simulink model "IMTrialSensorFinal"  (R2023b)
settings: Solver=VariableStepAuto  StartTime=0.0  StopTime=14  FixedStep=10e-6  RelTol=1e-3
settings Model: Creator=Aryasetya  LastModifiedBy=Aryasetya
settings ModelReferenceCC: EnableRefExpFcnMdlSchedulingChecks=on

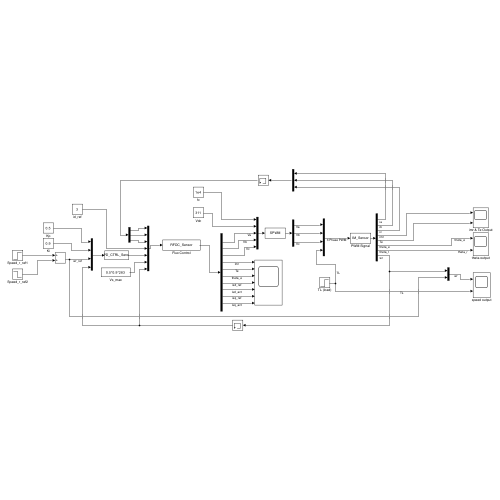
[thumbnail: Simulink's stored preview of the top-level diagram]
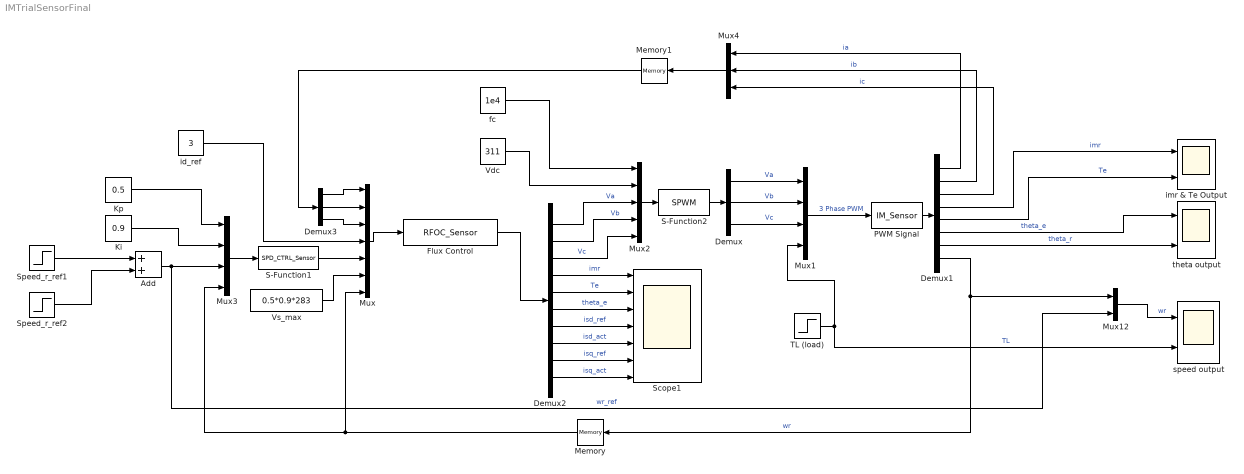
== system IMTrialSensorFinal ==
  Add : Sum
  Demux : Demux  Outputs=3
  Demux1 : Demux  Outputs=8
  Demux2 : Demux  Outputs=10
  Demux3 : Demux  Outputs=3
  Flux Control : S-Function  FunctionName=RFOC_Sensor  SFunctionDeploymentMode=off  EnableBusSupport=off
  Ki : Constant  Value=0.9
  Kp : Constant  Value=0.5
  Memory : Memory
  Memory1 : Memory
  Mux : Mux  Inputs=7
  Mux1 : Mux
  Mux12 : Mux  Inputs=2
  Mux2 : Mux  Inputs=5
  Mux3 : Mux
  Mux4 : Mux  Inputs=3
  PWM Signal : S-Function  FunctionName=IM_Sensor  SFunctionDeploymentMode=off  EnableBusSupport=off
  S-Function1 : S-Function  FunctionName=SPD_CTRL_Sensor  SFunctionDeploymentMode=off  EnableBusSupport=off
  S-Function2 : S-Function  FunctionName=SPWM  SFunctionDeploymentMode=off  EnableBusSupport=off
  Scope1 : Scope  NumInputPorts=7
  Speed_r_ref1 : Step  After=50  SampleTime=0
  Speed_r_ref2 : Step  Time=10  After=-20  SampleTime=0
  TL (load) : Step  Time=5  After=3  SampleTime=0
  Vdc : Constant  Value=311
  Vs_max : Constant  Value=0.5*0.9*283
  fc : Constant  Value=1e4
  id_ref : Constant  Value=3
  imr & Te Output : Scope  NumInputPorts=2
  speed output : Scope  NumInputPorts=2
  theta output : Scope  NumInputPorts=2
  wires:
  Mux1/1 -> PWM Signal/1  "3 Phase PWM"
  PWM Signal/1 -> Demux1/1
  Demux/3 -> Mux1/3  "Vc"
  Demux/2 -> Mux1/2  "Vb"
  Demux/1 -> Mux1/1  "Va"
  TL (load)/1 -> speed output/2, Mux1/4  "TL"
  Demux1/1 -> Mux4/1  "ia"
  Demux1/2 -> Mux4/2  "ib"
  Demux1/3 -> Mux4/3  "ic"
  Demux1/4 -> imr & Te Output/1  "imr"
  Demux1/5 -> imr & Te Output/2  "Te"
  Demux1/6 -> theta output/1  "theta_e"
  Flux Control/1 -> Demux2/1
  Mux/1 -> Flux Control/1
  S-Function1/1 -> Mux/5
  Mux3/1 -> S-Function1/1
  Ki/1 -> Mux3/2
  Kp/1 -> Mux3/1
  id_ref/1 -> Mux/4
  Demux3/2 -> Mux/2
  Demux3/1 -> Mux/1
  Demux3/3 -> Mux/3
  Mux4/1 -> Memory1/1
  Memory1/1 -> Demux3/1
  Vs_max/1 -> Mux/6
  Mux2/1 -> S-Function2/1
  Demux2/1 -> Mux2/3  "Va"
  Demux2/2 -> Mux2/4  "Vb"
  Demux2/3 -> Mux2/5  "Vc"
  Demux2/4 -> Scope1/1  "imr"
  Demux2/6 -> Scope1/3  "theta_e"
  Demux2/5 -> Scope1/2  "Te"
  Demux2/7 -> Scope1/4  "isd_ref"
  Demux2/8 -> Scope1/5  "isd_act"
  Demux2/9 -> Scope1/6  "isq_ref"
  Demux2/10 -> Scope1/7  "isq_act"
  S-Function2/1 -> Demux/1
  fc/1 -> Mux2/1
  Vdc/1 -> Mux2/2
  Speed_r_ref1/1 -> Add/1
  Add/1 -> Mux12/2, Mux3/3  "wr_ref"
  Speed_r_ref2/1 -> Add/2
  Demux1/8 -> Memory/1, Mux12/1  "wr"
  Demux1/7 -> theta output/2  "theta_r"
  Mux12/1 -> speed output/1  "wr"
  Memory/1 -> Mux3/4, Mux/7
